simulink model "my_sim_unsuccess"  (R2020a)
settings: Solver=VariableStepAuto  StartTime=0.0  StopTime=1  FixedStep=0.0000001  RelTol=1e-3
settings Model: Creator=td  LastModifiedBy=td
settings SolverCC: AlgebraicLoopSolver=LineSearch

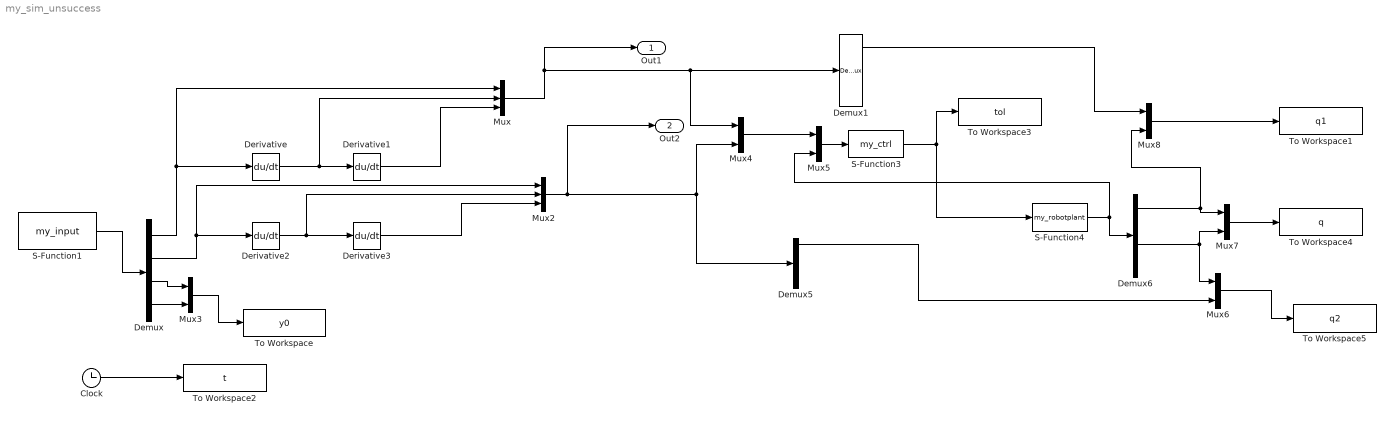
== system my_sim_unsuccess ==
  Clock : Clock
  Demux : Demux
  Demux1 : Demux  Outputs=3
  Demux5 : Demux  Outputs=3
  Demux6 : Demux
  Derivative{,1..3} (4 alike) : Derivative
  Mux : Mux  Inputs=3
  Mux2 : Mux  Inputs=3
  Mux{3..8} (6 alike) : Mux  Inputs=2
  S-Function1 : S-Function  FunctionName=my_input  SFunctionDeploymentMode=off  EnableBusSupport=off
  S-Function3 : S-Function  FunctionName=my_ctrl  SFunctionDeploymentMode=off  EnableBusSupport=off
  S-Function4 : S-Function  FunctionName=my_robotplant  SFunctionDeploymentMode=off  EnableBusSupport=off
  To Workspace : ToWorkspace  VariableName=y0  SaveFormat=Timeseries  SampleTime=-1
  To Workspace1 : ToWorkspace  VariableName=q1  SaveFormat=Timeseries  SampleTime=-1
  To Workspace2 : ToWorkspace  VariableName=t  SaveFormat=Timeseries  SampleTime=-1
  To Workspace3 : ToWorkspace  VariableName=tol  SaveFormat=Timeseries  SampleTime=-1
  To Workspace4 : ToWorkspace  VariableName=q  SaveFormat=Timeseries  SampleTime=-1
  To Workspace5 : ToWorkspace  VariableName=q2  SaveFormat=Timeseries  SampleTime=-1
  Out1 : Outport
  Out2 : Outport  Port=2
  wires:
  S-Function3/1 -> S-Function4/1, To Workspace3/1
  Mux2/1 -> Out2/1, Mux4/2, Demux5/1
  Mux6/1 -> To Workspace5/1
  Demux5/1 -> Mux6/2
  Mux5/1 -> S-Function3/1
  Mux7/1 -> To Workspace4/1
  Demux6/1 -> Mux8/2, Mux7/1
  Mux8/1 -> To Workspace1/1
  Mux4/1 -> Mux5/1
  Demux1/1 -> Mux8/1
  Mux/1 -> Out1/1, Mux4/1, Demux1/1
  S-Function4/1 -> Mux5/2, Demux6/1
  Demux/1 -> Mux/1, Derivative/1
  Demux/2 -> Mux2/1, Derivative2/1
  Derivative2/1 -> Mux2/2, Derivative3/1
  Derivative/1 -> Mux/2, Derivative1/1
  Derivative1/1 -> Mux/3
  Mux3/1 -> To Workspace/1
  Demux/4 -> Mux3/2
  Demux/3 -> Mux3/1
  S-Function1/1 -> Demux/1
  Derivative3/1 -> Mux2/3
  Clock/1 -> To Workspace2/1
  Demux6/3 -> Mux7/2, Mux6/1
